simulink model "full_Model"  (R2023b)
settings: Solver=ode15s  StartTime=0.0  StopTime=200  RelTol=1e-3
InitFcn:
  | clear all
  | clc
  | 
  | load('EnvironmentData.mat')
  | load('userMap.mat')
  | 
  | starty = 1;
  | startx = 1;
  | endy = 20;
  | endx = 20;
  | objy = [];
  | objx = [];
  | bally = 11;
  | ballx = 11;
  | 
  | objPos=[objx,objy];
  | ballPos=[11,11,0.54];
  | boxPos=[];
  | 
  | ManipulatorSetup
  | init_quad_new_leg_raibert_strategy_v2
  | transitionMode = [-1];
values from neighbouring files (symbols this model uses):
  body = rigidBody('tool')    [InverseKinematicsV2.m]
  tar1Len = 9    [EnvironmentData.mat]
  target = [1 2.44274045536 4.0666557818 4.62742644863 6.44502800895 8.36141317519 9.41392894318 10.3865588461 10.4 10.4 11.7644392896 13.2870590067 ... (34 elements, 17x2)]    [EnvironmentData.mat]
  tarLen = 17    [EnvironmentData.mat]
undefined symbols (not defined in the file or in its folder): planner
libraries: sim3dlib x33, sharedtransform x2, visionsinks x1, visionanalysis x1, visiongeotforms x1, sim3dcameralib x1
(part 5 of 7)

== matlab function full_Model/Controller/Quadruped movement Controller/state ==
  data: y output; t input
function y = statetest(t)
y=1;

if t > 85
    y = 3;
elseif t > 75
    y = 1;
elseif t > 60
    y = 2;
elseif t > 50
    y = 1;
elseif t > 35
    y = 3;
elseif t > 25
    y = 1;
elseif t > 10
    y = 2;
elseif t > 0
    y = 1;
end
